simulink model "my_model2c"  (R2022b)
settings: Solver=VariableStepAuto  StartTime=0.0  StopTime=10.0  RelTol=1e-3
values from neighbouring files (symbols this model uses):
  k = 1    [run_my_model2b.m]
  lower_sat = -1    [run_my_model2b.m]
  upper_sat = 1    [run_my_model2b.m]
undefined symbols (not defined in the file or in its folder): b
settings Model: Creator=royce  LastModifiedBy=royce
settings DataIOCC: ReturnWorkspaceOutputs=off

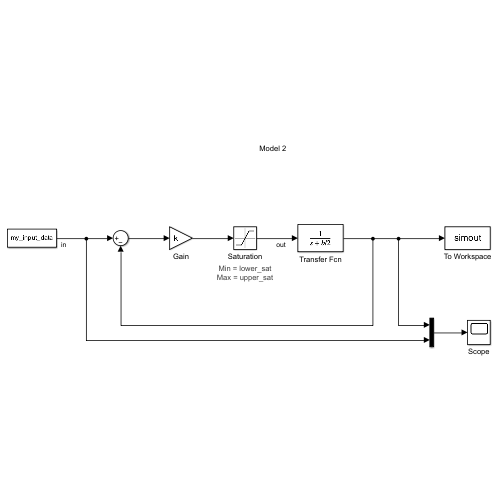
[thumbnail: Simulink's stored preview of the top-level diagram]
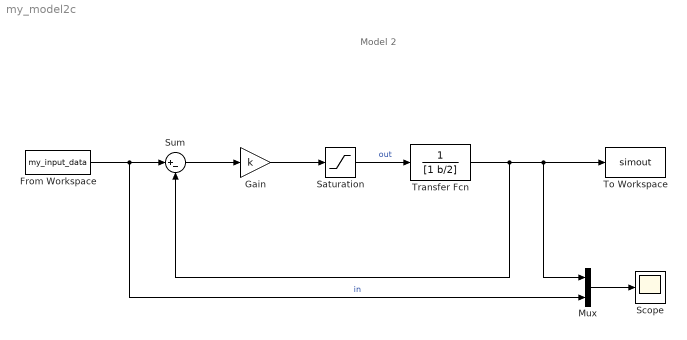
== system my_model2c ==
  note: Model 2
  From Workspace : FromWorkspace  VariableName=my_input_data
  Gain : Gain  Gain=k
  Mux : Mux  Inputs=2
  Saturation : Saturate  UpperLimit=upper_sat  LowerLimit=lower_sat
      settings: AttributesFormatString=|
      | Min = %<LowerLimit>
      | Max = %<UpperLimit>
  Scope : Scope
  Sum : Sum  Inputs=|+-
  To Workspace : ToWorkspace  VariableName=simout  SaveFormat=Timeseries  SampleTime=-1
  Transfer Fcn : TransferFcn  Denominator=[1 b/2]
  wires:
  From Workspace/1 -> Mux/2, Sum/1  "in"
  Gain/1 -> Saturation/1
  Saturation/1 -> Transfer Fcn/1  "out"
  Sum/1 -> Gain/1
  Mux/1 -> Scope/1
  Transfer Fcn/1 -> To Workspace/1, Mux/1, Sum/2
